simulink model "She_PWM"  (R2021a)
settings: Solver=FixedStepDiscrete  StartTime=0.0  StopTime=Tfinal  FixedStep=SampleTime  RelTol=1e-3
InitFcn:
  | param
values from neighbouring files (symbols this model uses):
  controlLoopTime = 6e-06    [param.m]
  fout = 50    [param.m]    (also in time_domain.m = 100; time_domain_2.m)
  fsw = 5e3    (= 5000)    [param.m]    (also in time_domain.m = 1000; time_domain_2.m = 1000)
  fsw_h = fsw+2*fout    (= 5100)    [param.m]    (also in time_domain.m = 1200)
  fsw_l = fsw-2*fout    (= 4900)    [param.m]    (also in time_domain.m = 800)
  ma = 0.9    [param.m]    (also in time_domain.m)
  mb = besselj(n,m*ma*pi/2)/(m*pi)    [param.m]    (also in time_domain_2.m = 2.*besselj(n,m*ma*pi/2)/(m*pi))
  phaseFout = 0    [param.m]
  SampleTime = 1/L1    (= 2.00080032013e-08)    [param.m]
libraries: spsFourierLib x16, spsTriangleGeneratorLib x5, eeGeneralControl x1, spspowerguiLib x1
settings Model: Creator=enes_  LastModifiedBy=enes_
settings SolverCC: AlgebraicLoopSolver=TrustRegion
settings DataIOCC: ReturnWorkspaceOutputs=off
settings DebuggingCC: SFMachineParentedDataDiag=warning  ArithmeticOperatorsInVariantConditions=warning
settings SFSimCC: SimUseLocalCustomCode=off  CustomCodeUndefinedFunction=UseInterfaceOnly
settings RTWCC: RTWUseLocalCustomCode=off

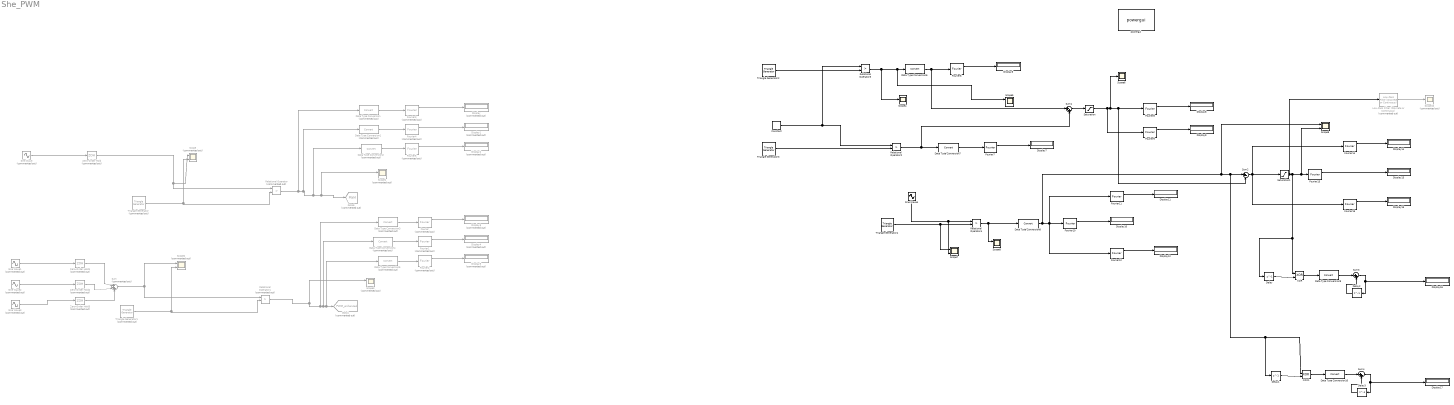
== system She_PWM ==
  Constant : Constant  Value=2*mb-1
  Data Type Conversion{,1..5} (6 alike) : DataTypeConversion  Commented=on
  Data Type Conversion{6..10} (5 alike) : DataTypeConversion
  Delay{,1..3} (4 alike) : Delay  DelayLength=1
  Display{,1..5} (6 alike) : Display  Commented=on
  Display{6..17} (12 alike) : Display
  Fourier : spsFourierLib/Fourier  Commented=on  Freq=50  n=(fsw/fout)-2  InInit=[0,0]  Ts=SampleTime
      settings: SourceProductBaseCode=PS
  Fourier1 : spsFourierLib/Fourier  Commented=on  Freq=50  n=(fsw/fout)  InInit=[0,0]  Ts=SampleTime
      settings: SourceProductBaseCode=PS
  Fourier10 : spsFourierLib/Fourier  Freq=fout  n=1  InInit=[0,0]  Ts=SampleTime
      settings: SourceProductBaseCode=PS
  Fourier11 : spsFourierLib/Fourier  Freq=fout  n=(fsw_l/fout)  InInit=[0,0]  Ts=SampleTime
      settings: SourceProductBaseCode=PS
  Fourier12 : spsFourierLib/Fourier  Freq=fout  n=(fsw_h/fout)  InInit=[0,0]  Ts=SampleTime
      settings: SourceProductBaseCode=PS
  Fourier13 : spsFourierLib/Fourier  Freq=fout  n=1  InInit=[0,0]  Ts=SampleTime
      settings: SourceProductBaseCode=PS
  Fourier14 : spsFourierLib/Fourier  Freq=fout  n=(fsw_l/fout)  InInit=[0,0]  Ts=SampleTime
      settings: SourceProductBaseCode=PS
  Fourier15 : spsFourierLib/Fourier  Freq=fout  n=(fsw_h/fout)  InInit=[0,0]  Ts=SampleTime
      settings: SourceProductBaseCode=PS
  Fourier2 : spsFourierLib/Fourier  Commented=on  Freq=50  n=(fsw/fout)+2  InInit=[0,0]  Ts=SampleTime
      settings: SourceProductBaseCode=PS
  Fourier3 : spsFourierLib/Fourier  Commented=on  Freq=50  n=(fsw/fout)-2  InInit=[0,0]  Ts=SampleTime
      settings: SourceProductBaseCode=PS
  Fourier4 : spsFourierLib/Fourier  Commented=on  Freq=50  n=(fsw/fout)  InInit=[0,0]  Ts=SampleTime
      settings: SourceProductBaseCode=PS
  Fourier5 : spsFourierLib/Fourier  Commented=on  Freq=50  n=(fsw/fout)+2  InInit=[0,0]  Ts=SampleTime
      settings: SourceProductBaseCode=PS
  Fourier6 : spsFourierLib/Fourier  Freq=fout  n=(fsw/fout)-2  InInit=[0,0]  Ts=SampleTime
      settings: SourceProductBaseCode=PS
  Fourier7 : spsFourierLib/Fourier  Freq=fout  n=(fsw/fout)+2  InInit=[0,0]  Ts=SampleTime
      settings: SourceProductBaseCode=PS
  Fourier8 : spsFourierLib/Fourier  Freq=fout  n=(fsw/fout)-2  InInit=[0,0]  Ts=SampleTime
      settings: SourceProductBaseCode=PS
  Fourier9 : spsFourierLib/Fourier  Freq=fout  n=(fsw/fout)+2  InInit=[0,0]  Ts=SampleTime
      settings: SourceProductBaseCode=PS
  Goto1 : Goto  Commented=on  GotoTag=PWM_enhanced  TagVisibility=global
  Goto6 : Goto  Commented=on  GotoTag=PWM  TagVisibility=global
  Low-Pass Filter (Discrete or Continuous) : eeGeneralControl/Low-Pass Filter (Discrete or Continuous)  Commented=on  K=1  T=0.0020  B=inf  A=-inf  init_option=Inherited from block input  x0=0  Ts=-1
  Relational Operator : RelationalOperator  Commented=on  Operator=>  OutDataTypeStr=boolean  RndMeth=Simplest
  Relational Operator1 : RelationalOperator  Commented=on  Operator=>  OutDataTypeStr=boolean  RndMeth=Simplest
  Relational Operator2 : RelationalOperator  Operator=>  OutDataTypeStr=boolean  RndMeth=Simplest
  Relational Operator3 : RelationalOperator  Operator=>  OutDataTypeStr=boolean  RndMeth=Simplest
  Relational Operator4 : RelationalOperator  Operator=>  OutDataTypeStr=boolean  RndMeth=Simplest
  Saturation : Saturate  UpperLimit=1  LowerLimit=0
  Saturation1 : Saturate  UpperLimit=1  LowerLimit=0
  Scope{,1..3} (4 alike) : Scope  Commented=on  NumInputPorts=2
  Scope10 : Scope  Commented=on
  Scope4 : Scope
  Scope{5,7..9} (4 alike) : Scope  NumInputPorts=2
  Scope6 : Scope
  Sine Wave : Sin  Commented=on  Amplitude=ma  Frequency=fout*2*pi  Phase=phaseFout  SampleTime=0
  Sine Wave1 : Sin  Commented=on  Amplitude=ma  Frequency=fout*2*pi  Phase=phaseFout  SampleTime=0
  Sine Wave2 : Sin  Commented=on  Amplitude=2*mb  Frequency=fsw_l*2*pi  Phase=-2*phaseFout  SampleTime=0
  Sine Wave3 : Sin  Commented=on  Amplitude=2*mb  Frequency=fsw_h*2*pi  Phase=2*phaseFout  SampleTime=0
  Sine Wave4 : Sin  Amplitude=ma  Frequency=fout*2*pi  SampleTime=0
  Sum : Sum  Commented=on  Inputs=|+++
  Sum1 : Sum  Inputs=|++
  Sum2 : Sum  Inputs=|+-
  Sum3 : Sum  Inputs=|++
  Sum4 : Sum  Inputs=|++
  Triangle Generator : spsTriangleGeneratorLib/Triangle Generator  Commented=on  Freq=fsw  Phase=0  Ts=0
  Triangle Generator1 : spsTriangleGeneratorLib/Triangle Generator  Commented=on  Freq=fsw  Phase=0  Ts=0
  Triangle Generator2 : spsTriangleGeneratorLib/Triangle Generator  Freq=fsw_l  Phase=0  Ts=0
  Triangle Generator3 : spsTriangleGeneratorLib/Triangle Generator  Freq=fsw_h  Phase=0  Ts=0
  Triangle Generator4 : spsTriangleGeneratorLib/Triangle Generator  Freq=fsw  Phase=0  Ts=0
  XOR : Logic  Operator=XOR  IconShape=distinctive  AllPortsSameDT=off  OutDataTypeStr=boolean
  XOR1 : Logic  Operator=XOR  IconShape=distinctive  AllPortsSameDT=off  OutDataTypeStr=boolean
  Zero-Order Hold{,1..3} (4 alike) : ZeroOrderHold  Commented=on  SampleTime=controlLoopTime
  powergui : spspowerguiLib/powergui  Priority=1  SimulationMode=Discrete  SampleTime=SampleTime  frequency=60  Iterations=50  frequencyindice=0  Pbase=100e6  ErrMax=1e-4  UnitsV=kV  UnitsW=MW  buscounter=0  FunctionMessages=off  echomessages=off  EnableUseOfTLC=off  CurrentSourceSwitches=off  DisableSnubberDevices=off  DisableRonSwitches=off  DisableVfSwitches=off  DisplayEquations=off  AutomaticDiscreteSolvers=off  SolverType=Tustin/Backward Euler (TBE)  Interpol=off  ExternalGateDelay=off  methode=off  Ts=100  x0status=blocks  SPID=on  SwTol=0  HookPort=off  NonlinearTolerance=1e-4  nMaxIteration=100  ContinueOnMaxIteration=off  RestoreLinks=warning  ResistiveCurrentMeasurement=off  Frange=[1e3:1e3:240e3]  Ylog=off  Xlog=on  ShowGrid=off  save=off  variable=ZData  structure=inputVoltage  ZoomFFT=off  StartTime=0.0  cycles=100  DisplayStyle=1  fundamental=80000  FreqAxis=off  MaxFrequency=240e3  frequencyindicesteady=1  RmsSteady=1  display=off
  wires:
  Triangle Generator/1 -> Relational Operator/2, Scope/2
  Sine Wave/1 -> Zero-Order Hold/1
  Zero-Order Hold/1 -> Relational Operator/1, Scope/1
  Sine Wave1/1 -> Zero-Order Hold1/1
  Triangle Generator1/1 -> Relational Operator1/2, Scope2/2
  Zero-Order Hold1/1 -> Sum/1
  Relational Operator1/1 -> Scope3/1, Data Type Conversion3/1, Data Type Conversion4/1, Data Type Conversion5/1, Goto1/1
  Sine Wave2/1 -> Zero-Order Hold2/1
  Sine Wave3/1 -> Zero-Order Hold3/1
  Zero-Order Hold2/1 -> Sum/2
  Zero-Order Hold3/1 -> Sum/3
  Sum/1 -> Relational Operator1/1, Scope2/1
  Relational Operator/1 -> Scope1/1, Goto6/1, Data Type Conversion2/1, Data Type Conversion1/1, Data Type Conversion/1
  Fourier3/1 -> Display/1
  Fourier4/1 -> Display1/1
  Fourier5/1 -> Display2/1
  Fourier/1 -> Display3/1
  Fourier1/1 -> Display4/1
  Fourier2/1 -> Display5/1
  Data Type Conversion/1 -> Fourier3/1
  Data Type Conversion1/1 -> Fourier4/1
  Data Type Conversion2/1 -> Fourier5/1
  Data Type Conversion3/1 -> Fourier/1
  Data Type Conversion4/1 -> Fourier1/1
  Data Type Conversion5/1 -> Fourier2/1
  Triangle Generator3/1 -> Relational Operator2/2
  Data Type Conversion6/1 -> Sum1/1, Fourier6/1
  Fourier6/1 -> Display6/1
  Data Type Conversion7/1 -> Fourier7/1
  Fourier7/1 -> Display7/1
  Constant/1 -> Relational Operator3/1, Relational Operator2/1
  Relational Operator2/1 -> Sum1/2, Data Type Conversion7/1
  Triangle Generator2/1 -> Relational Operator3/2
  Relational Operator3/1 -> Scope4/1, Scope5/1, Data Type Conversion6/1
  Fourier8/1 -> Display8/1
  Sum1/1 -> Saturation/1
  Fourier9/1 -> Display9/1
  Saturation/1 -> Sum2/2, Fourier8/1, Scope6/1, Fourier9/1
  Sine Wave4/1 -> Scope7/2, Relational Operator4/1
  Relational Operator4/1 -> Scope8/1, Data Type Conversion8/1
  Fourier10/1 -> Display10/1
  Triangle Generator4/1 -> Scope7/1, Relational Operator4/2
  Fourier11/1 -> Display11/1
  Fourier12/1 -> Display12/1
  Sum2/1 -> Fourier14/1, Fourier15/1, Saturation1/1
  Fourier15/1 -> Display15/1
  Fourier14/1 -> Display14/1
  Fourier13/1 -> Display13/1
  Saturation1/1 -> Low-Pass Filter (Discrete or Continuous)/1, Delay/1, XOR/1, Scope9/2, Fourier13/1
  Low-Pass Filter (Discrete or Continuous)/1 -> Scope10/1
  Delay/1 -> XOR/2
  Delay1/1 -> XOR1/2
  Data Type Conversion8/1 -> Scope9/1, XOR1/1, Delay1/1, Sum2/1, Fourier11/1, Fourier12/1, Fourier10/1
  XOR/1 -> Data Type Conversion9/1
  Delay2/1 -> Sum3/2
  XOR1/1 -> Data Type Conversion10/1
  Sum4/1 -> Display17/1, Delay3/1
  Delay3/1 -> Sum4/2
  Sum3/1 -> Display16/1, Delay2/1
  Data Type Conversion9/1 -> Sum3/1
  Data Type Conversion10/1 -> Sum4/1
